simulink model "untitled"  (R2017b)
settings: Solver=VariableStepAuto  StartTime=0.0  StopTime=10.0  RelTol=1e-6
settings Model: Creator=max  LastModifiedBy=max

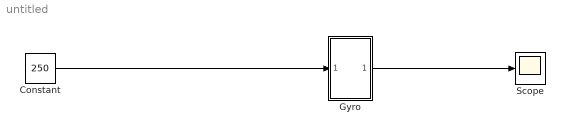
== system untitled ==
  Constant : Constant  Value=250
  Gyro : Subsystem
  Scope : Scope
  wires:
  Constant/1 -> Gyro/1(In1)
  Gyro/1(Out1) -> Scope/1

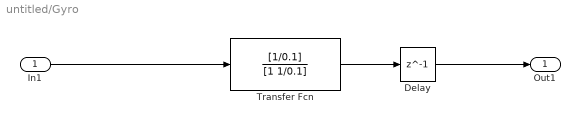
== system untitled/Gyro ==
  In1 : Inport
  Delay : Delay  DelayLength=1  SampleTime=1/400
  Transfer Fcn : TransferFcn  Numerator=[1/0.1]  Denominator=[1 1/0.1]
  Out1 : Outport
  wires:
  Transfer Fcn/1 -> Delay/1
  In1/1 -> Transfer Fcn/1
  Delay/1 -> Out1/1
